simulink model "LQR"  (R2022a)
settings: Solver=VariableStepAuto  StartTime=0.0  StopTime=12  RelTol=1e-3
values from neighbouring files (symbols this model uses):
  A = [0 0 0 0 0 1 0 0 0 0 0 2.495 ... (25 elements, 5x5)]    [var_lqr.mat]    (also in var_lqr2new.mat)
  B = [0 0 0 0 500]    [var_lqr.mat]    (also in var_lqr2new.mat)
  C = [1 0 0 0 0]    [var_lqr.mat]    (also in var_lqr2new.mat)
  K = [9.21954445729 6.42723435648 4.64240979432 0.441861242469 2.51459589145]    [var_lqr2new.mat]
undefined symbols (not defined in the file or in its folder): sigbuilder_block
libraries: simulink x2
settings Model: Creator=ngovi  LastModifiedBy=ngovi

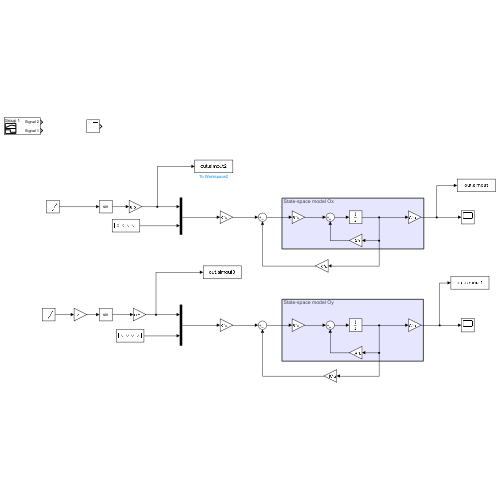
[thumbnail: Simulink's stored preview of the top-level diagram]
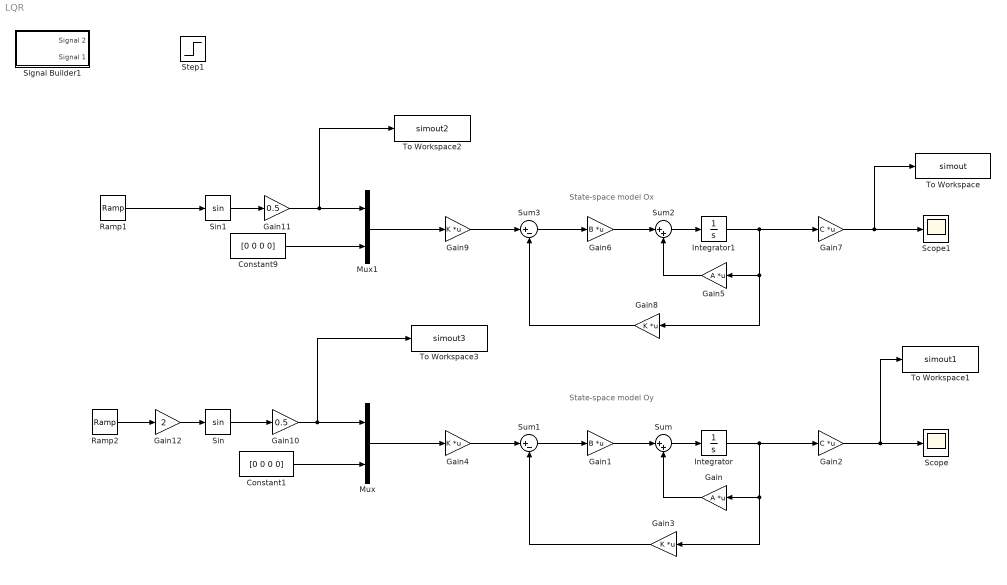
== system LQR ==
  note: State-space model Oy
  note: State-space model Ox
  Constant1 : Constant  Value=[0 0 0 0]
  Constant9 : Constant  Value=[0 0 0 0]
  Gain : Gain  Gain=A  Multiplication=Matrix(K*u)
  Gain1 : Gain  Gain=B  Multiplication=Matrix(K*u)
  Gain10 : Gain  Gain=0.5
  Gain11 : Gain  Gain=0.5
  Gain12 : Gain  Gain=2
  Gain2 : Gain  Gain=C  Multiplication=Matrix(K*u)
  Gain{3..4,8..9} (4 alike) : Gain  Gain=K  Multiplication=Matrix(K*u)
  Gain5 : Gain  Gain=A  Multiplication=Matrix(K*u)
  Gain6 : Gain  Gain=B  Multiplication=Matrix(K*u)
  Gain7 : Gain  Gain=C  Multiplication=Matrix(K*u)
  Integrator : Integrator
  Integrator1 : Integrator
  Mux : Mux  Inputs=2
  Mux1 : Mux  Inputs=2
  Ramp1 : simulink/Sources/Ramp  slope=2*pi/10  start=0  InitialOutput=0
  Ramp2 : simulink/Sources/Ramp  slope=2*pi/10  start=0  InitialOutput=0
  Scope : Scope
  Scope1 : Scope
  Signal Builder1 : Subsystem  Tag=STV Subsys  LoadFcn=sigbuilder_block('load');  StartFcn=sigbuilder_block('start');  StopFcn=sigbuilder_block('stop');  ClipboardFcn=sigbuilder_block('clipboard');  mask(Sigbuilder block){tuvar=[0:10]}
      mask help: Simulink:masks:SigbuilderBlock_MD
      mask init:
      | if ~strcmp(get_param(bdroot(gcbh),'SimulationStatus'),'stopped') tuvar = sigbuilder_block('maskInit'); end
      settings: CopyFcn=sigbuilder_block('copy');  DeleteFcn=sigbuilder_block('delete');  ModelCloseFcn=sigbuilder_block('modelClose');  PreSaveFcn=sigbuilder_block('preSave');  PauseFcn=sigbuilder_block('pause');  ContinueFcn=sigbuilder_block('continue');  NameChangeFcn=sigbuilder_block('namechange');  OpenFcn=sigbuilder_block('open',[0 36 1440 716.25 ]);  CloseFcn=sigbuilder_block('close');
      mask Display: plot(0, 0, 100, 100,[2, 2, 32, 32, 2], [68, 8, 8, 68, 68],[32, 2], [38, 38], [32, 19, 2],[53, 60, 44], [32, 17, 17, 2],[16, 16, 31, 31]);txt = getActiveGroup(gcbh);text(2, 100, txt,'verticalAlignment', 'top');
  Sin : Trigonometry
  Sin1 : Trigonometry
  Step1 : Step  Time=0  SampleTime=0
  Sum : Sum  Inputs=|++
  Sum1 : Sum  Inputs=|+-
  Sum2 : Sum  Inputs=|++
  Sum3 : Sum  Inputs=|+-
  To Workspace : ToWorkspace  VariableName=simout  SampleTime=-1
  To Workspace1 : ToWorkspace  VariableName=simout1  SampleTime=-1
  To Workspace2 : ToWorkspace  VariableName=simout2  SampleTime=-1
  To Workspace3 : ToWorkspace  VariableName=simout3  SampleTime=-1
  wires:
  Gain1/1 -> Sum/1
  Sum/1 -> Integrator/1
  Integrator/1 -> Gain3/1, Gain/1, Gain2/1
  Gain/1 -> Sum/2
  Sum1/1 -> Gain1/1
  Gain3/1 -> Sum1/2
  Gain2/1 -> To Workspace1/1, Scope/1
  Mux/1 -> Gain4/1
  Gain4/1 -> Sum1/1
  Ramp1/1 -> Sin1/1
  Gain9/1 -> Sum3/1
  Mux1/1 -> Gain9/1
  Gain7/1 -> To Workspace/1, Scope1/1
  Gain8/1 -> Sum3/2
  Sum3/1 -> Gain6/1
  Gain5/1 -> Sum2/2
  Integrator1/1 -> Gain7/1, Gain8/1, Gain5/1
  Sum2/1 -> Integrator1/1
  Gain6/1 -> Sum2/1
  Constant9/1 -> Mux1/2
  Constant1/1 -> Mux/2
  Sin/1 -> Gain10/1
  Ramp2/1 -> Gain12/1
  Sin1/1 -> Gain11/1
  Gain10/1 -> To Workspace3/1, Mux/1
  Gain11/1 -> To Workspace2/1, Mux1/1
  Gain12/1 -> Sin/1

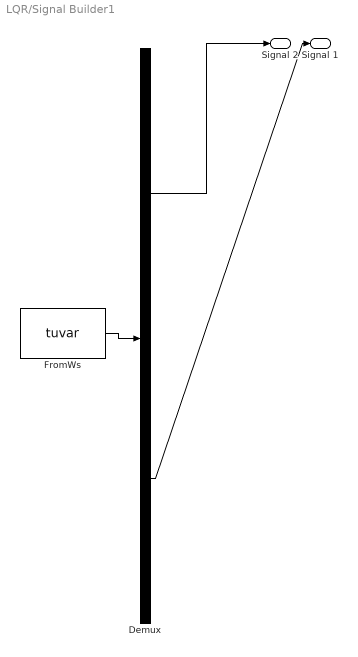
== system LQR/Signal Builder1 ==
  Demux : Demux  Tag=STV Demux  Outputs=2
      settings: DisplayOption=none
  FromWs : FromWorkspace  Tag=STV FromWs  VariableName=tuvar
      SigBuilderData=|
      | common.afterFinalStr = 'Extrapolate'
      | common.sampleTime = 0
      | dataSet.timeRange = [0 12]
      | dataSet.name = 'Group 1'
      | sbobj.Groups.Name = 'Group 1'
      | sbobj.Groups.Signals(1).Name = 'Signal 2'
      | sbobj.Groups.Signals(1).XData = [0 2 4 4 6 8 8 8.61 9.08 9.46 12]
      | sbobj.Groups.Signals(1).YData = [49.8 49.8 49.8 -50 -50 -50 50 50 50 50 50]
      | sbobj.Groups.Signals(2).Name = 'Signal 1'
      | sbobj.Groups.Signals(2).XData = [0 2.01 2.01 3.56 6 6 7.16 8.32 9.13 10.01 10.01 12]
      | sbobj.Groups.Signals(2).YData = [0 0 50 50 50 -50 -50 -50 -50 -50 45.5 45.5]
      | sbobj.Groups.TimeRange = [0 12]
  Signal 2 : Outport  Tag=STV Outport
  Signal 1 : Outport  Tag=STV Outport  Port=2
  wires:
  FromWs/1 -> Demux/1
  Demux/1 -> Signal 2/1
  Demux/2 -> Signal 1/1
